simulink model "PILnewH"  (R2021a)
settings: Solver=FixedStepAuto  StartTime=0.0  StopTime=41.24  FixedStep=0.001  RelTol=1e-3  EnableMultiTasking=on
values from neighbouring files (symbols this model uses):
  den_lpf_d = den_lpf20    [Mainframe_init.m]    (also in load_autopilot.m)
  Emulated_FCC_IO_Delay = 7    [Mainframe_init.m]
  Enable_Gyros = 0    [Mainframe_init.m]
  Enable_INS = 0    [Mainframe_init.m]
  num_lpf_d = num_lpf20    [Mainframe_init.m]    (also in load_autopilot.m)
undefined symbols (not defined in the file or in its folder): act_dmp, act_omega, Actuator, Aerodynamics, aMode, Autopilot, AUX, c_b_WGS, c_be, c_flat, c_grav, c_h_geop0, c_h_geope, c_pa0, c_pe, c_r0, c_rot, c_rsma, c_Tmp0, d_siB_0, d_siB_max, d_siB_min, dd_siB_max, dd_siB_min, dev, DiscIntNeverNeededParam, e_pa, e_Tmp, Earth, fin_maxrate, flag_I_act_switch, flag_I_aero_switch, flag_I_flat, flag_I_gravity_switch, flag_I_rot, hcr, HIL_Data, JMMM_0, JMMM_e, JSPB_e, lat_0, lon_0, Mass_Props, mB_0, mM_0, mM_e, National_Instruments, pBII_0, PCIe, pMPB, pNPB, propellant_kg, prp_FBPB, prp_mdot, prp_T, pSPB, pwm_output1, qEG_0, qIB_0, qIE_0 ... (+29)
libraries: simulink x31, simulink_extras x24, aerolibcommonsys x4, px4lib x2, custom_blocks x1, pil_lib x1, aerolibtransform2 x1, sldrtlib x1, aerolibnav x1
(part 7 of 15)

== system PILnewH/Non-linear Flight Dynamic Model/Extract States/Assemble_States_Bus1/Three-axis Inertial Measurement Unit3/Three-axis Accelerometer/w x (w x d) ==
  "p q r " : Inport
  distance : Inport  Port=2
  w x (w x d) : Subsystem  mask(CrossProduct){aMode=aMode}
      mask help: shared_aeroblks:sharedaeroblkutil:blockCrossProductDesc
      mask init:
      | if aerosharedtest(gcb)
      |     aerosharedicon('shared');
      | else
      |     sharedautoicon('shared');
      | end
      mask Help: eval('if license(''test'',''Aerospace_Blockset'')aerosharedhelp(''threebythree_cross_product'');elseif license(''test'',''Powertrain_Blockset'')sharedautohelp(''threebythree_cross_product'');end')
      mask Display:
      | text(.5,.5,'Cross\nProduct\nC = AxB', ...
      | 	'HorizontalAlignment','Center',...
      | 	'VerticalAlignment','middle')
  w x d : Subsystem  mask(CrossProduct){aMode=aMode}
      mask help: shared_aeroblks:sharedaeroblkutil:blockCrossProductDesc
      mask init:
      | if aerosharedtest(gcb)
      |     aerosharedicon('shared');
      | else
      |     sharedautoicon('shared');
      | end
      mask Help: eval('if license(''test'',''Aerospace_Blockset'')aerosharedhelp(''threebythree_cross_product'');elseif license(''test'',''Powertrain_Blockset'')sharedautohelp(''threebythree_cross_product'');end')
      mask Display:
      | text(.5,.5,'Cross\nProduct\nC = AxB', ...
      | 	'HorizontalAlignment','Center',...
      | 	'VerticalAlignment','middle')
  w x ( w x d) : Outport  VectorParamsAs1DForOutWhenUnconnected=off
  wires:
  "p q r "/1 -> w x (w x d)/1(A), w x d/1(A)
  w x d/1(C) -> w x (w x d)/2(B)
  distance/1 -> w x d/2(B)
  w x (w x d)/1(C) -> w x ( w x d)/1

== system PILnewH/Non-linear Flight Dynamic Model/Extract States/Assemble_States_Bus1/Three-axis Inertial Measurement Unit3/Three-axis Accelerometer/wdot x d ==
  A : Inport
  B : Inport  Port=2
  "A " : InportShadow
  "B " : InportShadow  Port=2
  Subsystem : Subsystem
  Subsystem1 : Subsystem
  Sum : Sum  Inputs=+|-  InputSameDT=on  SaturateOnIntegerOverflow=on  OutDataTypeStr=Inherit: Same as first input
  C : Outport  VectorParamsAs1DForOutWhenUnconnected=off
  wires:
  Subsystem1/1(Out1) -> Sum/2
  Subsystem/1(Out1) -> Sum/1
  A/1 -> Subsystem/1(A)
  B/1 -> Subsystem/2(B)
  Sum/1 -> C/1
  "A "/1 -> Subsystem1/1(A)
  "B "/1 -> Subsystem1/2(B)

== system PILnewH/Non-linear Flight Dynamic Model/Extract States/Assemble_States_Bus1/Three-axis Inertial Measurement Unit3/Three-axis Gyroscope/Dynamics ==
  p q r : Inport
  Constant : Constant  Value=dtype_g
  No Dynamics : Subsystem
  Second-order Dynamics : Subsystem  mask(ContinuousFilter){wn=w_g, zn=z_g}
      mask prompts: wn "Natural frequency:"; zn "Damping ratio:"
      mask init:
      | aeroicon('aeroblk');
  Switch : Switch  Threshold=0.5
  "p q r " : Outport  VectorParamsAs1DForOutWhenUnconnected=off
  wires:
  p q r/1 -> Second-order Dynamics/1(In), No Dynamics/1(In1)
  No Dynamics/1(Out1) -> Switch/3
  Second-order Dynamics/1(Out) -> Switch/1
  Switch/1 -> "p q r "/1
  Constant/1 -> Switch/2

== system PILnewH/Non-linear Flight Dynamic Model/GRM_Airframe/aerodynamics/aerodynamic_via_lookup/calc_aero_coefficients/CLL_TLU ==
  alpha_deg : Inport
  beta_deg : Inport  Port=2
  dele_deg : Inport  Port=3
  dela_deg : Inport  Port=4
  delr_deg : Inport  Port=5
  p_ND_rps : Inport  Port=6
  1-D Lookup Table : Lookup_n-D  NumberOfTableDimensions=1  BreakpointsForDimension1=Aerodynamics.alpha_bkpts_ind1  Table=Aerodynamics.CLL_alpha  ExtrapMethod=Clip  UseLastTableValue=on  InternalRulePriority=Speed  RndMeth=Simplest  InputSameDT=on
      settings: AttributesFormatString=|
      | %<Table>
      | %<BreakpointsForDimension1>
  1-D Lookup Table1 : Lookup_n-D  NumberOfTableDimensions=1  BreakpointsForDimension1=Aerodynamics.beta_bkpts_ind1  Table=Aerodynamics.CLL_beta  ExtrapMethod=Clip  UseLastTableValue=on  InternalRulePriority=Speed  RndMeth=Simplest  InputSameDT=on
      settings: AttributesFormatString=|
      | %<Table>
      | %<BreakpointsForDimension1>
  2-D Lookup Table : Lookup_n-D  BreakpointsForDimension1=Aerodynamics.dele_inc_bkpts_ind1  BreakpointsForDimension2=Aerodynamics.dele_inc_bkpts_ind2  Table=Aerodynamics.CLL_dele_inc  ExtrapMethod=Clip  UseLastTableValue=on  InternalRulePriority=Speed  RndMeth=Simplest  InputSameDT=on
      settings: InputPortMap=u0,u1
      settings: AttributesFormatString=|
      | %<Table>
      | %<BreakpointsForDimension1>
      | %<BreakpointsForDimension2>
  2-D Lookup Table1 : Lookup_n-D  BreakpointsForDimension1=Aerodynamics.dela_inc_bkpts_ind1  BreakpointsForDimension2=Aerodynamics.dela_inc_bkpts_ind2  Table=Aerodynamics.CLL_dela_inc  ExtrapMethod=Clip  UseLastTableValue=on  InternalRulePriority=Speed  RndMeth=Simplest  InputSameDT=on
      settings: InputPortMap=u0,u1
      settings: AttributesFormatString=|
      | %<Table>
      | %<BreakpointsForDimension1>
      | %<BreakpointsForDimension2>
  2-D Lookup Table2 : Lookup_n-D  BreakpointsForDimension1=Aerodynamics.delr_inc_bkpts_ind1  BreakpointsForDimension2=Aerodynamics.delr_inc_bkpts_ind2  Table=Aerodynamics.CLL_delr_inc  ExtrapMethod=Clip  UseLastTableValue=on  InternalRulePriority=Speed  RndMeth=Simplest  InputSameDT=on
      settings: InputPortMap=u0,u1
      settings: AttributesFormatString=|
      | %<Table>
      | %<BreakpointsForDimension1>
      | %<BreakpointsForDimension2>
  Constant : Constant  Value=Aerodynamics.CLL_bias
      settings: AttributesFormatString=%<Value>
  Gain : Gain  Gain=Aerodynamics.CLL_scale
      settings: AttributesFormatString=%<Gain>
  Gain2 : Gain  Gain=Aerodynamics.CLL_p
      settings: AttributesFormatString=%<Gain>
  Sum1 : Sum  Inputs=+++++
  Sum2 : Sum
  Sum3 : Sum  Inputs=|++
  alpha_deg D1 : InportShadow
  alpha_deg D2 : InportShadow
  beta_deg D1 : InportShadow  Port=2
  CLL : Outport
  wires:
  p_ND_rps/1 -> Gain2/1
  Gain2/1 -> Sum1/5
  Gain/1 -> Sum3/1
  2-D Lookup Table2/1 -> Sum1/4  "CLL_delr"
  1-D Lookup Table/1 -> Sum2/1
  2-D Lookup Table1/1 -> Sum1/3  "CLL_dela"
  beta_deg/1 -> 1-D Lookup Table1/1
  1-D Lookup Table1/1 -> Sum2/2
  2-D Lookup Table/1 -> Sum1/2  "CLL_dele"
  dele_deg/1 -> 2-D Lookup Table/2
  alpha_deg D1/1 -> 2-D Lookup Table/1
  beta_deg D1/1 -> 2-D Lookup Table2/1
  dela_deg/1 -> 2-D Lookup Table1/2
  alpha_deg/1 -> 1-D Lookup Table/1
  alpha_deg D2/1 -> 2-D Lookup Table1/1
  delr_deg/1 -> 2-D Lookup Table2/2
  Sum2/1 -> Sum1/1  "CLL_0"
  Constant/1 -> Sum3/2
  Sum1/1 -> Gain/1
  Sum3/1 -> CLL/1  "CLL_B"

== system PILnewH/Non-linear Flight Dynamic Model/GRM_Airframe/aerodynamics/aerodynamic_via_lookup/calc_aero_coefficients/CLM_TLU ==
  alpha_deg : Inport
  beta_deg : Inport  Port=2
  dele_deg : Inport  Port=3
  dela_deg : Inport  Port=4
  delr_deg : Inport  Port=5
  q_ND_rps : Inport  Port=6
  1-D Lookup Table : Lookup_n-D  NumberOfTableDimensions=1  BreakpointsForDimension1=Aerodynamics.alpha_bkpts_ind1  Table=Aerodynamics.CLM_alpha  ExtrapMethod=Clip  UseLastTableValue=on  InternalRulePriority=Speed  RndMeth=Simplest  InputSameDT=on
      settings: AttributesFormatString=|
      | %<Table>
      | %<BreakpointsForDimension1>
  1-D Lookup Table1 : Lookup_n-D  NumberOfTableDimensions=1  BreakpointsForDimension1=Aerodynamics.beta_bkpts_ind1  Table=Aerodynamics.CLM_beta  ExtrapMethod=Clip  UseLastTableValue=on  InternalRulePriority=Speed  RndMeth=Simplest  InputSameDT=on
      settings: AttributesFormatString=|
      | %<Table>
      | %<BreakpointsForDimension1>
  2-D Lookup Table : Lookup_n-D  BreakpointsForDimension1=Aerodynamics.dele_inc_bkpts_ind1  BreakpointsForDimension2=Aerodynamics.dele_inc_bkpts_ind2  Table=Aerodynamics.CLM_dele_inc  ExtrapMethod=Clip  UseLastTableValue=on  InternalRulePriority=Speed  RndMeth=Simplest  InputSameDT=on
      settings: InputPortMap=u0,u1
      settings: AttributesFormatString=|
      | %<Table>
      | %<BreakpointsForDimension1>
      | %<BreakpointsForDimension2>
  2-D Lookup Table1 : Lookup_n-D  BreakpointsForDimension1=Aerodynamics.dela_inc_bkpts_ind1  BreakpointsForDimension2=Aerodynamics.dela_inc_bkpts_ind2  Table=Aerodynamics.CLM_dela_inc  ExtrapMethod=Clip  UseLastTableValue=on  InternalRulePriority=Speed  RndMeth=Simplest  InputSameDT=on
      settings: InputPortMap=u0,u1
      settings: AttributesFormatString=|
      | %<Table>
      | %<BreakpointsForDimension1>
      | %<BreakpointsForDimension2>
  2-D Lookup Table2 : Lookup_n-D  BreakpointsForDimension1=Aerodynamics.delr_inc_bkpts_ind1  BreakpointsForDimension2=Aerodynamics.delr_inc_bkpts_ind2  Table=Aerodynamics.CLM_delr_inc  ExtrapMethod=Clip  UseLastTableValue=on  InternalRulePriority=Speed  RndMeth=Simplest  InputSameDT=on
      settings: InputPortMap=u0,u1
      settings: AttributesFormatString=|
      | %<Table>
      | %<BreakpointsForDimension1>
      | %<BreakpointsForDimension2>
  Constant : Constant  Value=Aerodynamics.CLM_bias
      settings: AttributesFormatString=%<Value>
  Gain : Gain  Gain=Aerodynamics.CLM_scale
      settings: AttributesFormatString=%<Gain>
  Gain2 : Gain  Gain=Aerodynamics.CLM_q
      settings: AttributesFormatString=%<Gain>
  Sum1 : Sum  Inputs=+++++
  Sum2 : Sum
  Sum3 : Sum  Inputs=|++
  alpha_deg D1 : InportShadow
  alpha_deg D2 : InportShadow
  beta_deg D1 : InportShadow  Port=2
  CLM : Outport
  wires:
  q_ND_rps/1 -> Gain2/1
  Gain2/1 -> Sum1/5
  Sum3/1 -> CLM/1  "CLM_B"
  delr_deg/1 -> 2-D Lookup Table2/2
  alpha_deg D2/1 -> 2-D Lookup Table1/1
  dela_deg/1 -> 2-D Lookup Table1/2
  alpha_deg/1 -> 1-D Lookup Table/1
  beta_deg D1/1 -> 2-D Lookup Table2/1
  alpha_deg D1/1 -> 2-D Lookup Table/1
  1-D Lookup Table1/1 -> Sum2/2
  dele_deg/1 -> 2-D Lookup Table/2
  2-D Lookup Table/1 -> Sum1/2  "CLM_dele"
  2-D Lookup Table1/1 -> Sum1/3  "CLM_dela"
  beta_deg/1 -> 1-D Lookup Table1/1
  2-D Lookup Table2/1 -> Sum1/4  "CLM_delr"
  Sum2/1 -> Sum1/1  "CLM_0"
  1-D Lookup Table/1 -> Sum2/1
  Sum1/1 -> Gain/1
  Constant/1 -> Sum3/2
  Gain/1 -> Sum3/1

== system PILnewH/Non-linear Flight Dynamic Model/GRM_Airframe/aerodynamics/aerodynamic_via_lookup/calc_aero_coefficients/CLN_TLU ==
  alpha_deg : Inport
  beta_deg : Inport  Port=2
  dele_deg : Inport  Port=3
  dela_deg : Inport  Port=4
  delr_deg : Inport  Port=5
  r_ND_rps : Inport  Port=6
  1-D Lookup Table : Lookup_n-D  NumberOfTableDimensions=1  BreakpointsForDimension1=Aerodynamics.alpha_bkpts_ind1  Table=Aerodynamics.CLN_alpha  ExtrapMethod=Clip  UseLastTableValue=on  InternalRulePriority=Speed  RndMeth=Simplest  InputSameDT=on
      settings: AttributesFormatString=|
      | %<Table>
      | %<BreakpointsForDimension1>
  1-D Lookup Table1 : Lookup_n-D  NumberOfTableDimensions=1  BreakpointsForDimension1=Aerodynamics.beta_bkpts_ind1  Table=Aerodynamics.CLN_beta  ExtrapMethod=Clip  UseLastTableValue=on  InternalRulePriority=Speed  RndMeth=Simplest  InputSameDT=on
      settings: AttributesFormatString=|
      | %<Table>
      | %<BreakpointsForDimension1>
  2-D Lookup Table : Lookup_n-D  BreakpointsForDimension1=Aerodynamics.dele_inc_bkpts_ind1  BreakpointsForDimension2=Aerodynamics.dele_inc_bkpts_ind2  Table=Aerodynamics.CLN_dele_inc  ExtrapMethod=Clip  UseLastTableValue=on  InternalRulePriority=Speed  RndMeth=Simplest  InputSameDT=on
      settings: InputPortMap=u0,u1
      settings: AttributesFormatString=|
      | %<Table>
      | %<BreakpointsForDimension1>
      | %<BreakpointsForDimension2>
  2-D Lookup Table1 : Lookup_n-D  BreakpointsForDimension1=Aerodynamics.dela_inc_bkpts_ind1  BreakpointsForDimension2=Aerodynamics.dela_inc_bkpts_ind2  Table=Aerodynamics.CLN_dela_inc  ExtrapMethod=Clip  UseLastTableValue=on  InternalRulePriority=Speed  RndMeth=Simplest  InputSameDT=on
      settings: InputPortMap=u0,u1
      settings: AttributesFormatString=|
      | %<Table>
      | %<BreakpointsForDimension1>
      | %<BreakpointsForDimension2>
  2-D Lookup Table2 : Lookup_n-D  BreakpointsForDimension1=Aerodynamics.delr_inc_bkpts_ind1  BreakpointsForDimension2=Aerodynamics.delr_inc_bkpts_ind2  Table=Aerodynamics.CLN_delr_inc  ExtrapMethod=Clip  UseLastTableValue=on  InternalRulePriority=Speed  RndMeth=Simplest  InputSameDT=on
      settings: InputPortMap=u0,u1
      settings: AttributesFormatString=|
      | %<Table>
      | %<BreakpointsForDimension1>
      | %<BreakpointsForDimension2>
  Constant : Constant  Value=Aerodynamics.CLN_bias
      settings: AttributesFormatString=%<Value>
  Gain : Gain  Gain=Aerodynamics.CLN_scale
      settings: AttributesFormatString=%<Gain>
  Gain2 : Gain  Gain=Aerodynamics.CLN_r
      settings: AttributesFormatString=%<Gain>
  Sum1 : Sum  Inputs=+++++
  Sum2 : Sum
  Sum3 : Sum  Inputs=|++
  alpha_deg D1 : InportShadow
  alpha_deg D2 : InportShadow
  beta_deg D1 : InportShadow  Port=2
  CLN : Outport
  wires:
  r_ND_rps/1 -> Gain2/1
  Sum3/1 -> CLN/1  "CLN_B"
  beta_deg/1 -> 1-D Lookup Table1/1
  1-D Lookup Table/1 -> Sum2/1
  2-D Lookup Table2/1 -> Sum1/4  "CLN_delr"
  Sum2/1 -> Sum1/1  "CLN_0"
  alpha_deg D1/1 -> 2-D Lookup Table/1
  beta_deg D1/1 -> 2-D Lookup Table2/1
  dele_deg/1 -> 2-D Lookup Table/2
  alpha_deg D2/1 -> 2-D Lookup Table1/1
  2-D Lookup Table1/1 -> Sum1/3  "CLN_dela"
  alpha_deg/1 -> 1-D Lookup Table/1
  dela_deg/1 -> 2-D Lookup Table1/2
  Gain2/1 -> Sum1/5
  1-D Lookup Table1/1 -> Sum2/2
  delr_deg/1 -> 2-D Lookup Table2/2
  2-D Lookup Table/1 -> Sum1/2  "CLN_dele"
  Sum1/1 -> Gain/1
  Constant/1 -> Sum3/2
  Gain/1 -> Sum3/1

== system PILnewH/Non-linear Flight Dynamic Model/GRM_Airframe/aerodynamics/aerodynamic_via_lookup/calc_aero_coefficients/CX_TLU ==
  alpha_deg : Inport
  beta_deg : Inport  Port=2
  dele_deg : Inport  Port=3
  dela_deg : Inport  Port=4
  delr_deg : Inport  Port=5
  2-D Lookup Table : Lookup_n-D  BreakpointsForDimension1=Aerodynamics.alpha_beta_bkpts_ind1  BreakpointsForDimension2=Aerodynamics.alpha_beta_bkpts_ind2  Table=Aerodynamics.CX_alpha_beta  ExtrapMethod=Clip  UseLastTableValue=on  InternalRulePriority=Speed  RndMeth=Simplest  InputSameDT=on
      settings: InputPortMap=u0,u1
      settings: AttributesFormatString=|
      | %<Table>
      | %<BreakpointsForDimension1>
      | %<BreakpointsForDimension2>
  2-D Lookup Table1 : Lookup_n-D  BreakpointsForDimension1=Aerodynamics.dele_inc_bkpts_ind1  BreakpointsForDimension2=Aerodynamics.dele_inc_bkpts_ind2  Table=Aerodynamics.CX_dele_inc  ExtrapMethod=Clip  UseLastTableValue=on  InternalRulePriority=Speed  RndMeth=Simplest  InputSameDT=on
      settings: InputPortMap=u0,u1
      settings: AttributesFormatString=|
      | %<Table>
      | %<BreakpointsForDimension1>
      | %<BreakpointsForDimension2>
  2-D Lookup Table2 : Lookup_n-D  BreakpointsForDimension1=Aerodynamics.dela_inc_bkpts_ind1  BreakpointsForDimension2=Aerodynamics.dela_inc_bkpts_ind2  Table=Aerodynamics.CX_dela_inc  ExtrapMethod=Clip  UseLastTableValue=on  InternalRulePriority=Speed  RndMeth=Simplest  InputSameDT=on
      settings: InputPortMap=u0,u1
      settings: AttributesFormatString=|
      | %<Table>
      | %<BreakpointsForDimension1>
      | %<BreakpointsForDimension2>
  2-D Lookup Table3 : Lookup_n-D  BreakpointsForDimension1=Aerodynamics.delr_inc_bkpts_ind1  BreakpointsForDimension2=Aerodynamics.delr_inc_bkpts_ind2  Table=Aerodynamics.CX_delr_inc  ExtrapMethod=Clip  UseLastTableValue=on  InternalRulePriority=Speed  RndMeth=Simplest  InputSameDT=on
      settings: InputPortMap=u0,u1
      settings: AttributesFormatString=|
      | %<Table>
      | %<BreakpointsForDimension1>
      | %<BreakpointsForDimension2>
  Constant : Constant  Value=Aerodynamics.CX_bias
      settings: AttributesFormatString=%<Value>
  Gain : Gain  Gain=Aerodynamics.CX_scale
      settings: AttributesFormatString=%<Gain>
  Sum : Sum  Inputs=++++
  Sum1 : Sum  Inputs=|++
  alpha_deg D1 : InportShadow
  alpha_deg D2 : InportShadow
  beta_deg D1 : InportShadow  Port=2
  CX : Outport
  wires:
  Sum/1 -> Gain/1
  2-D Lookup Table1/1 -> Sum/2  "CX_dele"
  2-D Lookup Table2/1 -> Sum/3  "CX_dela"
  2-D Lookup Table/1 -> Sum/1  "CX_0"
  alpha_deg/1 -> 2-D Lookup Table/1
  beta_deg/1 -> 2-D Lookup Table/2
  alpha_deg D1/1 -> 2-D Lookup Table1/1
  dele_deg/1 -> 2-D Lookup Table1/2
  dela_deg/1 -> 2-D Lookup Table2/2
  2-D Lookup Table3/1 -> Sum/4  "CX_delr"
  delr_deg/1 -> 2-D Lookup Table3/2
  alpha_deg D2/1 -> 2-D Lookup Table2/1
  beta_deg D1/1 -> 2-D Lookup Table3/1
  Constant/1 -> Sum1/2
  Gain/1 -> Sum1/1
  Sum1/1 -> CX/1  "CX_B"

== system PILnewH/Non-linear Flight Dynamic Model/GRM_Airframe/aerodynamics/aerodynamic_via_lookup/calc_aero_coefficients/CY_TLU ==
  alpha_deg : Inport
  beta_deg : Inport  Port=2
  dele_deg : Inport  Port=3
  dela_deg : Inport  Port=4
  delr_deg : Inport  Port=5
  1-D Lookup Table : Lookup_n-D  NumberOfTableDimensions=1  BreakpointsForDimension1=Aerodynamics.alpha_bkpts_ind1  Table=Aerodynamics.CY_alpha  ExtrapMethod=Clip  UseLastTableValue=on  InternalRulePriority=Speed  RndMeth=Simplest  InputSameDT=on
      settings: AttributesFormatString=|
      | %<Table>
      | %<BreakpointsForDimension1>
  1-D Lookup Table1 : Lookup_n-D  NumberOfTableDimensions=1  BreakpointsForDimension1=Aerodynamics.beta_bkpts_ind1  Table=Aerodynamics.CY_beta  ExtrapMethod=Clip  UseLastTableValue=on  InternalRulePriority=Speed  RndMeth=Simplest  InputSameDT=on
      settings: AttributesFormatString=|
      | %<Table>
      | %<BreakpointsForDimension1>
  2-D Lookup Table : Lookup_n-D  BreakpointsForDimension1=Aerodynamics.dele_inc_bkpts_ind1  BreakpointsForDimension2=Aerodynamics.dele_inc_bkpts_ind2  Table=Aerodynamics.CY_dele_inc  ExtrapMethod=Clip  UseLastTableValue=on  InternalRulePriority=Speed  RndMeth=Simplest  InputSameDT=on
      settings: InputPortMap=u0,u1
      settings: AttributesFormatString=|
      | %<Table>
      | %<BreakpointsForDimension1>
      | %<BreakpointsForDimension2>
  2-D Lookup Table1 : Lookup_n-D  BreakpointsForDimension1=Aerodynamics.dela_inc_bkpts_ind1  BreakpointsForDimension2=Aerodynamics.dela_inc_bkpts_ind2  Table=Aerodynamics.CY_dela_inc  ExtrapMethod=Clip  UseLastTableValue=on  InternalRulePriority=Speed  RndMeth=Simplest  InputSameDT=on
      settings: InputPortMap=u0,u1
      settings: AttributesFormatString=|
      | %<Table>
      | %<BreakpointsForDimension1>
      | %<BreakpointsForDimension2>
  2-D Lookup Table2 : Lookup_n-D  BreakpointsForDimension1=Aerodynamics.delr_inc_bkpts_ind1  BreakpointsForDimension2=Aerodynamics.delr_inc_bkpts_ind2  Table=Aerodynamics.CY_delr_inc  ExtrapMethod=Clip  UseLastTableValue=on  InternalRulePriority=Speed  RndMeth=Simplest  InputSameDT=on
      settings: InputPortMap=u0,u1
      settings: AttributesFormatString=|
      | %<Table>
      | %<BreakpointsForDimension1>
      | %<BreakpointsForDimension2>
  Constant : Constant  Value=Aerodynamics.CY_bias
      settings: AttributesFormatString=%<Value>
  Gain : Gain  Gain=Aerodynamics.CY_scale
      settings: AttributesFormatString=%<Gain>
  Sum : Sum  Inputs=++++
  Sum1 : Sum
  Sum2 : Sum  Inputs=|++
  alpha_deg D1 : InportShadow
  alpha_deg D2 : InportShadow
  beta_deg D1 : InportShadow  Port=2
  CY : Outport
  wires:
  Sum2/1 -> CY/1  "CY_B"
  beta_deg/1 -> 1-D Lookup Table1/1
  1-D Lookup Table/1 -> Sum1/1
  1-D Lookup Table1/1 -> Sum1/2
  alpha_deg/1 -> 1-D Lookup Table/1
  alpha_deg D1/1 -> 2-D Lookup Table/1
  alpha_deg D2/1 -> 2-D Lookup Table1/1
  2-D Lookup Table2/1 -> Sum/4  "CY_delr"
  delr_deg/1 -> 2-D Lookup Table2/2
  2-D Lookup Table1/1 -> Sum/3  "CY_dela"
  2-D Lookup Table/1 -> Sum/2  "CY_dele"
  beta_deg D1/1 -> 2-D Lookup Table2/1
  dela_deg/1 -> 2-D Lookup Table1/2
  dele_deg/1 -> 2-D Lookup Table/2
  Sum1/1 -> Sum/1  "CY_0"
  Gain/1 -> Sum2/1
  Constant/1 -> Sum2/2
  Sum/1 -> Gain/1

== system PILnewH/Non-linear Flight Dynamic Model/GRM_Airframe/aerodynamics/aerodynamic_via_lookup/calc_aero_coefficients/CZ_TLU ==
  alpha_deg : Inport
  beta_deg : Inport  Port=2
  dele_deg : Inport  Port=3
  dela_deg : Inport  Port=4
  delr_deg : Inport  Port=5
  1-D Lookup Table : Lookup_n-D  NumberOfTableDimensions=1  BreakpointsForDimension1=Aerodynamics.alpha_bkpts_ind1  Table=Aerodynamics.CZ_alpha  ExtrapMethod=Clip  UseLastTableValue=on  InternalRulePriority=Speed  RndMeth=Simplest  InputSameDT=on
      settings: AttributesFormatString=|
      | %<Table>
      | %<BreakpointsForDimension1>
  1-D Lookup Table1 : Lookup_n-D  NumberOfTableDimensions=1  BreakpointsForDimension1=Aerodynamics.beta_bkpts_ind1  Table=Aerodynamics.CZ_beta  ExtrapMethod=Clip  UseLastTableValue=on  InternalRulePriority=Speed  RndMeth=Simplest  InputSameDT=on
      settings: AttributesFormatString=|
      | %<Table>
      | %<BreakpointsForDimension1>
  2-D Lookup Table : Lookup_n-D  BreakpointsForDimension1=Aerodynamics.dele_inc_bkpts_ind1  BreakpointsForDimension2=Aerodynamics.dele_inc_bkpts_ind2  Table=Aerodynamics.CZ_dele_inc  ExtrapMethod=Clip  UseLastTableValue=on  InternalRulePriority=Speed  RndMeth=Simplest  InputSameDT=on
      settings: InputPortMap=u0,u1
      settings: AttributesFormatString=|
      | %<Table>
      | %<BreakpointsForDimension1>
      | %<BreakpointsForDimension2>
  2-D Lookup Table1 : Lookup_n-D  BreakpointsForDimension1=Aerodynamics.dela_inc_bkpts_ind1  BreakpointsForDimension2=Aerodynamics.dela_inc_bkpts_ind2  Table=Aerodynamics.CZ_dela_inc  ExtrapMethod=Clip  UseLastTableValue=on  InternalRulePriority=Speed  RndMeth=Simplest  InputSameDT=on
      settings: InputPortMap=u0,u1
      settings: AttributesFormatString=|
      | %<Table>
      | %<BreakpointsForDimension1>
      | %<BreakpointsForDimension2>
  2-D Lookup Table2 : Lookup_n-D  BreakpointsForDimension1=Aerodynamics.delr_inc_bkpts_ind1  BreakpointsForDimension2=Aerodynamics.delr_inc_bkpts_ind2  Table=Aerodynamics.CZ_delr_inc  ExtrapMethod=Clip  UseLastTableValue=on  InternalRulePriority=Speed  RndMeth=Simplest  InputSameDT=on
      settings: InputPortMap=u0,u1
      settings: AttributesFormatString=|
      | %<Table>
      | %<BreakpointsForDimension1>
      | %<BreakpointsForDimension2>
  Constant : Constant  Value=Aerodynamics.CZ_bias
      settings: AttributesFormatString=%<Value>
  Gain : Gain  Gain=Aerodynamics.CZ_scale
      settings: AttributesFormatString=%<Gain>
  Sum : Sum  Inputs=++++
  Sum1 : Sum
  Sum2 : Sum  Inputs=|++
  alpha_deg D1 : InportShadow
  alpha_deg D2 : InportShadow
  beta_deg D1 : InportShadow  Port=2
  CZ : Outport
  wires:
  dele_deg/1 -> 2-D Lookup Table/2
  dela_deg/1 -> 2-D Lookup Table1/2
  beta_deg D1/1 -> 2-D Lookup Table2/1
  2-D Lookup Table/1 -> Sum/2  "CZ_dele"
  2-D Lookup Table1/1 -> Sum/3  "CZ_dela"
  delr_deg/1 -> 2-D Lookup Table2/2
  2-D Lookup Table2/1 -> Sum/4  "CZ_delr"
  alpha_deg D2/1 -> 2-D Lookup Table1/1
  alpha_deg D1/1 -> 2-D Lookup Table/1
  alpha_deg/1 -> 1-D Lookup Table/1
  1-D Lookup Table1/1 -> Sum1/2
  1-D Lookup Table/1 -> Sum1/1
  Sum1/1 -> Sum/1  "CZ_0"
  beta_deg/1 -> 1-D Lookup Table1/1
  Sum2/1 -> CZ/1  "CZ_B"
  Constant/1 -> Sum2/2
  Gain/1 -> Sum2/1
  Sum/1 -> Gain/1

== system PILnewH/Non-linear Flight Dynamic Model/GRM_Airframe/aerodynamics/aerodynamic_via_lookup/calc_aero_for_mom/create_pAPB ==
  Constant : Constant  Value=Aerodynamics.xcg
      settings: AttributesFormatString=%<Value>
  Constant3 : Constant  Value=0
  Gain : Gain  Gain=-1
  Vector Concatenate : Concatenate  NumInputs=3
  pAPB : Outport  VectorParamsAs1DForOutWhenUnconnected=off
  wires:
  Constant3/1 -> Vector Concatenate/3, Vector Concatenate/2
  Gain/1 -> Vector Concatenate/1
  Constant/1 -> Gain/1
  Vector Concatenate/1 -> pAPB/1  "pAPB"

== system PILnewH/Non-linear Flight Dynamic Model/GRM_Airframe/aerodynamics/aerodynamic_via_lookup/calc_aero_for_mom/cross_product ==
  note: Outputs [size]:
      |
      | r1 x r2  [3x1]
  note: Inputs [size]:
      |
      | r1 [3x1]
      | r2 [3x1]
  r1 : Inport
  r2 : Inport  Port=2
  Demux2 : Demux  Outputs=[1;1;1]
      settings: DisplayOption=none
  Demux3 : Demux  Outputs=[1;1;1]
      settings: DisplayOption=none
  Product{2..7} (6 alike) : Product  InputSameDT=on  RndMeth=Zero  SaturateOnIntegerOverflow=on  OutDataTypeStr=Inherit: Same as first input
  Sum : Sum  Inputs=+-  InputSameDT=on  SaturateOnIntegerOverflow=on  OutDataTypeStr=Inherit: Same as first input
  Sum1 : Sum  Inputs=+-  InputSameDT=on  SaturateOnIntegerOverflow=on  OutDataTypeStr=Inherit: Same as first input
  Sum2 : Sum  Inputs=+-  InputSameDT=on  SaturateOnIntegerOverflow=on  OutDataTypeStr=Inherit: Same as first input
  Vector Concatenate : Concatenate  NumInputs=3
  r1_x_r2 : Outport  PortDimensions=[3,1]  VectorParamsAs1DForOutWhenUnconnected=off
  wires:
  Demux2/2 -> Product2/1, Product7/1
  Demux3/3 -> Product5/2, Product2/2
  Demux3/2 -> Product6/2, Product3/2
  Demux2/3 -> Product3/1, Product4/1
  Demux3/1 -> Product7/2, Product4/2
  Demux2/1 -> Product6/1, Product5/1
  Product2/1 -> Sum/1
  Product3/1 -> Sum/2
  Product4/1 -> Sum1/1
  Product5/1 -> Sum1/2
  Product6/1 -> Sum2/1
  Product7/1 -> Sum2/2
  Sum/1 -> Vector Concatenate/1
  Sum1/1 -> Vector Concatenate/2
  Sum2/1 -> Vector Concatenate/3
  r1/1 -> Demux2/1
  r2/1 -> Demux3/1
  Vector Concatenate/1 -> r1_x_r2/1

== system PILnewH/Non-linear Flight Dynamic Model/GRM_Airframe/aerodynamics/aerodynamic_via_lookup/calc_aero_for_mom/launch_rail ==
  hBE : Inport
  FBAB_c : Inport  Port=2
  Constant1 : Constant  Value=flag_I_aero_switch
  Constant3 : Constant  Value=0
  Subtract : Sum  Inputs=++-
  Switch : Switch  Criteria=u2 > Threshold  Threshold=0.05
  Vector Concatenate : Concatenate  NumInputs=3
  initial_altitude : Subsystem
  FBAB : Outport  VectorParamsAs1DForOutWhenUnconnected=off
  wires:
  Constant1/1 -> Subtract/2
  hBE/1 -> Subtract/1
  Subtract/1 -> Switch/2
  Constant3/1 -> Vector Concatenate/1, Vector Concatenate/2, Vector Concatenate/3
  Switch/1 -> FBAB/1  "FBAB"
  Vector Concatenate/1 -> Switch/3
  FBAB_c/1 -> Switch/1
  initial_altitude/1(hBE_0) -> Subtract/3

== system PILnewH/Non-linear Flight Dynamic Model/GRM_Airframe/aerodynamics/aerodynamic_via_lookup/calc_aero_for_mom/launch_rail1 ==
  hBE : Inport
  MBAB_c : Inport  Port=2
  Constant1 : Constant  Value=flag_I_aero_switch
  Constant3 : Constant  Value=0
  Subtract : Sum  Inputs=++-
  Switch : Switch  Criteria=u2 > Threshold  Threshold=0.05
  Vector Concatenate : Concatenate  NumInputs=3
  initial_altitude : Subsystem
  MBAB : Outport  VectorParamsAs1DForOutWhenUnconnected=off
  wires:
  initial_altitude/1(hBE_0) -> Subtract/3
  MBAB_c/1 -> Switch/1
  Vector Concatenate/1 -> Switch/3
  Switch/1 -> MBAB/1  "MBAB"
  Constant3/1 -> Vector Concatenate/3, Vector Concatenate/2, Vector Concatenate/1
  Subtract/1 -> Switch/2
  hBE/1 -> Subtract/1
  Constant1/1 -> Subtract/2

== system PILnewH/Non-linear Flight Dynamic Model/GRM_Airframe/environment/WGS84_Gravitation/WGS84_2_ECEF/WGS84 Transformation Parameter  ==
  phi : Inport
  Add2 : Sum  Inputs=+-
  Divide : Product  Inputs=**
  Divide1 : Product  Inputs=**
  Divide2 : Product  Inputs=**
  Divide3 : Product  Inputs=/*
  Sqrt : Sqrt  SaturateOnIntegerOverflow=on
  Subsystem : Subsystem
  Trigonometric Function : Trigonometry
  "WGS84 Semi-major Axis, [m]" : Constant  Value=c_rsma
  "WGS84 Semi-minor Axis, [m]" : Constant  Value=c_b_WGS
  a3 : Constant
  N : Outport  VectorParamsAs1DForOutWhenUnconnected=off
  e : Outport  Port=2  VectorParamsAs1DForOutWhenUnconnected=off
  wires:
  "WGS84 Semi-minor Axis, [m]"/1 -> Subsystem/1(b)  "c_b_WGS"
  "WGS84 Semi-major Axis, [m]"/1 -> Subsystem/2(a), Divide3/2  "c_rsma"
  Divide1/1 -> Divide2/1  "sin(phi)^2"
  Divide3/1 -> N/1  "N"
  Sqrt/1 -> Divide3/1
  a3/1 -> Add2/1
  Divide2/1 -> Add2/2
  Trigonometric Function/1 -> Divide1/2, Divide1/1
  Divide/1 -> Divide2/2  "e^2"
  Subsystem/1(e) -> e/1, Divide/2, Divide/1
  Add2/1 -> Sqrt/1
  phi/1 -> Trigonometric Function/1

== system PILnewH/Non-linear Flight Dynamic Model/GRM_Airframe/environment/atmosphere_static_ISO_2533/tmp_and_pressure_ISO_2533/static_Temperature ==
  Tmp_ref : Inport
  h_geop : Inport  Port=2
  h_geop_ref : Inport  Port=3
  Add : Sum
  Product : Product
  Subtract : Sum  Inputs=+-
  Tmp_gradient_tropo : Constant  Value=c_be
  Tmp : Outport  VectorParamsAs1DForOutWhenUnconnected=off
  wires:
  Subtract/1 -> Product/2
  Tmp_gradient_tropo/1 -> Product/1
  Product/1 -> Add/2
  Add/1 -> Tmp/1  "Tmp"
  Tmp_ref/1 -> Add/1
  h_geop/1 -> Subtract/1
  h_geop_ref/1 -> Subtract/2

== system PILnewH/Non-linear Flight Dynamic Model/GRM_Airframe/environment/atmosphere_static_ISO_2533/tmp_and_pressure_ISO_2533/static_pressure ==
  h_geop_ref : Inport
  h_geop : Inport  Port=2
  Tmp_ref : Inport  Port=3
  pa_ref : Inport  Port=4
  Add : Sum
  Constant1 : Constant
  Divide : Product  Inputs=*/*
  Math Function : Math  Operator=pow  SignedPower=on  SaturateOnIntegerOverflow=on
  Product : Product
  Subtract : Sum  Inputs=-+
  Tmp_gradient_tropo : Constant  Value=c_be
  pressure_exponent : Constant  Value=c_pe
  pa : Outport  VectorParamsAs1DForOutWhenUnconnected=off
  wires:
  pressure_exponent/1 -> Math Function/2
  h_geop/1 -> Subtract/2
  Divide/1 -> Add/2
  h_geop_ref/1 -> Subtract/1
  Tmp_ref/1 -> Divide/2
  Add/1 -> Math Function/1
  pa_ref/1 -> Product/2
  Math Function/1 -> Product/1
  Subtract/1 -> Divide/1
  Constant1/1 -> Add/1
  Product/1 -> pa/1  "pa"
  Tmp_gradient_tropo/1 -> Divide/3

== system PILnewH/Non-linear Flight Dynamic Model/GRM_Airframe/gravity/launch_rail/initial_altitude/trafo_E_to_geodetic ==
  note: Outputs [size]:
      |
      | geodetic longitude [1]
      | geodetic latitude [1]
      | geodetic altitude [1]
  note: Inputs [size]:
      |
      | position_E [3]
  pBEE : Inport
  Geodetic_altitude : Subsystem
  Geodetic_latitude : Subsystem
  Selector1 : Selector  IndexMode=Zero-based  InputPortWidth=3  IndexOptions=Index vector (dialog)  Indices=1  OutputSizes=1
  Selector2 : Selector  IndexMode=Zero-based  InputPortWidth=3  IndexOptions=Index vector (dialog)  Indices=0  OutputSizes=1
  Trigonometric Function1 : Trigonometry  Operator=atan2
  c_flat : Constant  Value=c_flat
  c_rsma : Constant  Value=c_rsma
  lon : Outport  VectorParamsAs1DForOutWhenUnconnected=off
  lat : Outport  Port=2  VectorParamsAs1DForOutWhenUnconnected=off
  alt : Outport  Port=3  VectorParamsAs1DForOutWhenUnconnected=off
  wires:
  c_flat/1 -> Geodetic_altitude/3(c_flat), Geodetic_latitude/3(c_flat)  "c_flat"
  c_rsma/1 -> Geodetic_latitude/2(c_rsma), Geodetic_altitude/2(c_rsma)  "c_rsma"
  Selector1/1 -> Trigonometric Function1/1  "pBEE_y"
  Selector2/1 -> Trigonometric Function1/2  "pBEE_x"
  Geodetic_latitude/1(lat) -> Geodetic_altitude/4(lat), lat/1
  Geodetic_altitude/1(alt) -> alt/1
  Trigonometric Function1/1 -> lon/1  "lon"
  pBEE/1 -> Selector1/1, Selector2/1, Geodetic_latitude/1(pBEE), Geodetic_altitude/1(pBEE)  "pBEE"

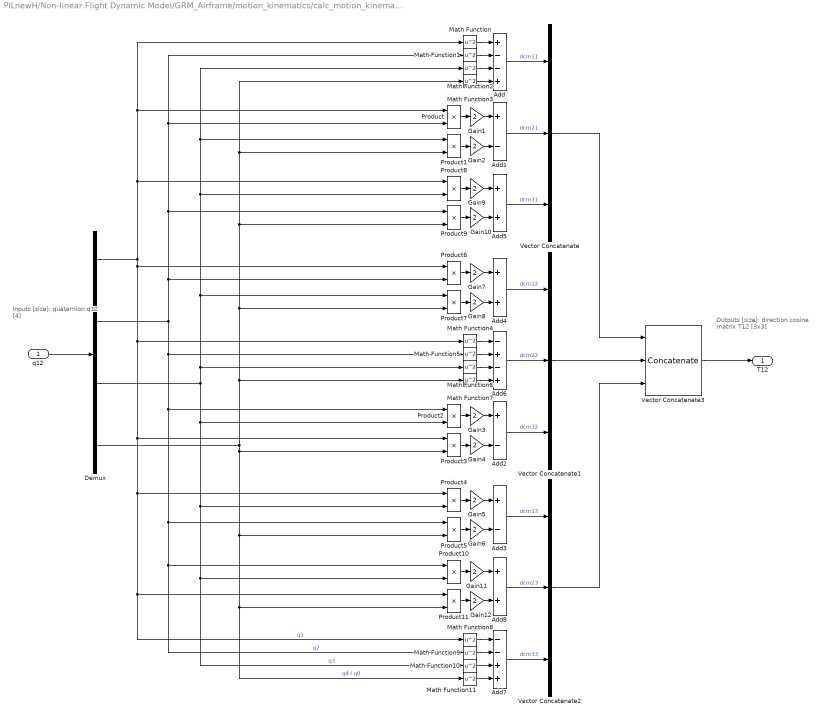
== system PILnewH/Non-linear Flight Dynamic Model/GRM_Airframe/motion_kinematics/calc_motion_kinematics/calc_transformation_matrix/T12_from_q1 ==
  note: Inputs [size]:
      |
      | quaternion q12 [4]
  note: Outputs [size]:
      |
      | direction cosine matrix T12 [3x3]
  q12 : Inport  PortDimensions=4
  Add : Sum  Inputs=+--+
  Add1 : Sum  Inputs=+-
  Add2 : Sum  Inputs=+-
  Add3 : Sum  Inputs=+-
  Add4 : Sum
  Add5 : Sum
  Add6 : Sum  Inputs=-+-+
  Add7 : Sum  Inputs=--++
  Add8 : Sum
  Demux : Demux
  Gain{1..12} (12 alike) : Gain  Gain=2
  Math Function{,1..11} (12 alike) : Math  Operator=square  SignedPower=on  SaturateOnIntegerOverflow=on
  Product{,1..11} (12 alike) : Product
  Vector Concatenate : Concatenate  NumInputs=3
  Vector Concatenate1 : Concatenate  NumInputs=3
  Vector Concatenate2 : Concatenate  NumInputs=3
  Vector Concatenate3 : Concatenate  NumInputs=3  Mode=Multidimensional array  ConcatenateDimension=2
  T12 : Outport  PortDimensions=[3 3]  VectorParamsAs1DForOutWhenUnconnected=off
  wires:
  Product10/1 -> Gain11/1
  Product11/1 -> Gain12/1
  Gain11/1 -> Add8/1
  Gain12/1 -> Add8/2
  Math Function8/1 -> Add7/1
  Math Function9/1 -> Add7/2
  Math Function11/1 -> Add7/4
  Math Function10/1 -> Add7/3
  Math Function4/1 -> Add6/1
  Math Function5/1 -> Add6/2
  Math Function7/1 -> Add6/4
  Math Function6/1 -> Add6/3
  Product8/1 -> Gain9/1
  Product9/1 -> Gain10/1
  Gain9/1 -> Add5/1
  Gain10/1 -> Add5/2
  Product6/1 -> Gain7/1
  Product7/1 -> Gain8/1
  Gain7/1 -> Add4/1
  Gain8/1 -> Add4/2
  Product4/1 -> Gain5/1
  Product5/1 -> Gain6/1
  Gain5/1 -> Add3/1
  Gain6/1 -> Add3/2
  Product2/1 -> Gain3/1
  Product3/1 -> Gain4/1
  Gain3/1 -> Add2/1
  Gain4/1 -> Add2/2
  Gain2/1 -> Add1/2
  Gain1/1 -> Add1/1
  Product1/1 -> Gain2/1
  Product/1 -> Gain1/1
  Math Function3/1 -> Add/4
  Math Function2/1 -> Add/3
  Math Function1/1 -> Add/2
  Math Function/1 -> Add/1
  Add7/1 -> Vector Concatenate2/3  "dcm33"
  Add8/1 -> Vector Concatenate2/2  "dcm23"
  Add3/1 -> Vector Concatenate2/1  "dcm13"
  Add2/1 -> Vector Concatenate1/3  "dcm32"
  Add6/1 -> Vector Concatenate1/2  "dcm22"
  Add4/1 -> Vector Concatenate1/1  "dcm12"
  Add5/1 -> Vector Concatenate/3  "dcm31"
  Add1/1 -> Vector Concatenate/2  "dcm21"
  Add/1 -> Vector Concatenate/1  "dcm11"
  Vector Concatenate1/1 -> Vector Concatenate3/2
  Vector Concatenate2/1 -> Vector Concatenate3/3
  Vector Concatenate/1 -> Vector Concatenate3/1
  Vector Concatenate3/1 -> T12/1
  Demux/4 -> Product3/2, Product11/2, Math Function11/1, Product5/2, Math Function3/1, Product1/2, Product9/2, Product7/2, Math Function7/1  "q4 / q0"
  Demux/3 -> Math Function2/1, Product1/1, Product8/2, Product7/1, Math Function6/1, Product10/2, Math Function10/1, Product4/2, Product2/2  "q3"
  Demux/2 -> Math Function1/1, Product/2, Product9/1, Product6/2, Math Function5/1, Math Function9/1, Product10/1, Product5/1, Product2/1  "q2"
  Demux/1 -> Product6/1, Math Function4/1, Math Function8/1, Product11/1, Product4/1, Product3/1, Math Function/1, Product/1, Product8/1  "q1"
  q12/1 -> Demux/1

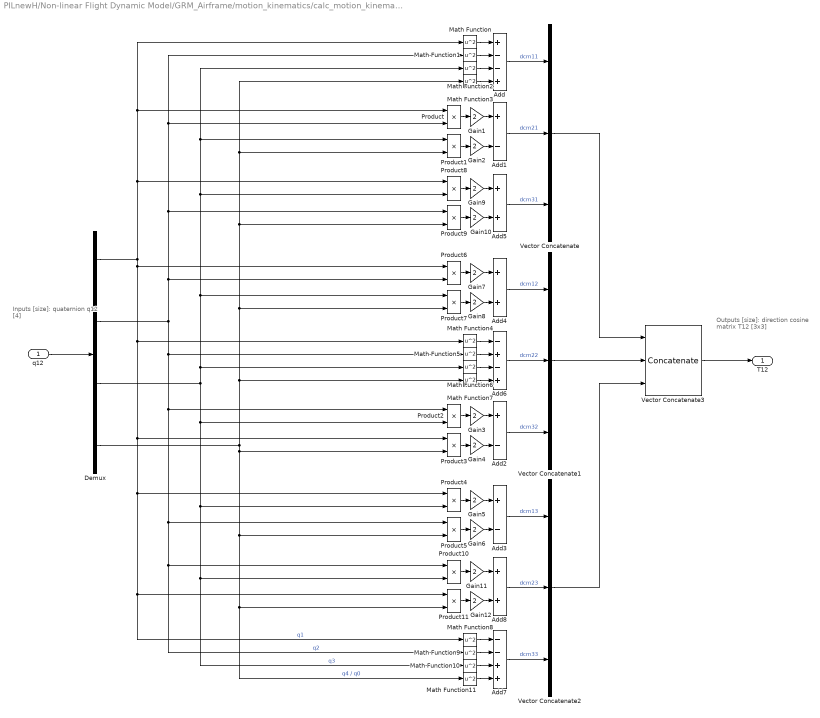
== system PILnewH/Non-linear Flight Dynamic Model/GRM_Airframe/motion_kinematics/calc_motion_kinematics/calc_transformation_matrix/T12_from_q12 ==
  note: Inputs [size]:
      |
      | quaternion q12 [4]
  note: Outputs [size]:
      |
      | direction cosine matrix T12 [3x3]
  q12 : Inport  PortDimensions=4
  Add : Sum  Inputs=+--+
  Add1 : Sum  Inputs=+-
  Add2 : Sum  Inputs=+-
  Add3 : Sum  Inputs=+-
  Add4 : Sum
  Add5 : Sum
  Add6 : Sum  Inputs=-+-+
  Add7 : Sum  Inputs=--++
  Add8 : Sum
  Demux : Demux
  Gain{1..12} (12 alike) : Gain  Gain=2
  Math Function{,1..11} (12 alike) : Math  Operator=square  SignedPower=on  SaturateOnIntegerOverflow=on
  Product{,1..11} (12 alike) : Product
  Vector Concatenate : Concatenate  NumInputs=3
  Vector Concatenate1 : Concatenate  NumInputs=3
  Vector Concatenate2 : Concatenate  NumInputs=3
  Vector Concatenate3 : Concatenate  NumInputs=3  Mode=Multidimensional array  ConcatenateDimension=2
  T12 : Outport  PortDimensions=[3 3]  VectorParamsAs1DForOutWhenUnconnected=off
  wires:
  Product10/1 -> Gain11/1
  Product11/1 -> Gain12/1
  Gain11/1 -> Add8/1
  Gain12/1 -> Add8/2
  Math Function8/1 -> Add7/1
  Math Function9/1 -> Add7/2
  Math Function11/1 -> Add7/4
  Math Function10/1 -> Add7/3
  Math Function4/1 -> Add6/1
  Math Function5/1 -> Add6/2
  Math Function7/1 -> Add6/4
  Math Function6/1 -> Add6/3
  Product8/1 -> Gain9/1
  Product9/1 -> Gain10/1
  Gain9/1 -> Add5/1
  Gain10/1 -> Add5/2
  Product6/1 -> Gain7/1
  Product7/1 -> Gain8/1
  Gain7/1 -> Add4/1
  Gain8/1 -> Add4/2
  Product4/1 -> Gain5/1
  Product5/1 -> Gain6/1
  Gain5/1 -> Add3/1
  Gain6/1 -> Add3/2
  Product2/1 -> Gain3/1
  Product3/1 -> Gain4/1
  Gain3/1 -> Add2/1
  Gain4/1 -> Add2/2
  Gain2/1 -> Add1/2
  Gain1/1 -> Add1/1
  Product1/1 -> Gain2/1
  Product/1 -> Gain1/1
  Math Function3/1 -> Add/4
  Math Function2/1 -> Add/3
  Math Function1/1 -> Add/2
  Math Function/1 -> Add/1
  Add7/1 -> Vector Concatenate2/3  "dcm33"
  Add8/1 -> Vector Concatenate2/2  "dcm23"
  Add3/1 -> Vector Concatenate2/1  "dcm13"
  Add2/1 -> Vector Concatenate1/3  "dcm32"
  Add6/1 -> Vector Concatenate1/2  "dcm22"
  Add4/1 -> Vector Concatenate1/1  "dcm12"
  Add5/1 -> Vector Concatenate/3  "dcm31"
  Add1/1 -> Vector Concatenate/2  "dcm21"
  Add/1 -> Vector Concatenate/1  "dcm11"
  Vector Concatenate1/1 -> Vector Concatenate3/2
  Vector Concatenate2/1 -> Vector Concatenate3/3
  Vector Concatenate/1 -> Vector Concatenate3/1
  Vector Concatenate3/1 -> T12/1
  Demux/4 -> Product3/2, Product11/2, Math Function11/1, Product5/2, Math Function3/1, Product1/2, Product9/2, Product7/2, Math Function7/1  "q4 / q0"
  Demux/3 -> Math Function2/1, Product1/1, Product8/2, Product7/1, Math Function6/1, Product10/2, Math Function10/1, Product4/2, Product2/2  "q3"
  Demux/2 -> Math Function1/1, Product/2, Product9/1, Product6/2, Math Function5/1, Math Function9/1, Product10/1, Product5/1, Product2/1  "q2"
  Demux/1 -> Product6/1, Math Function4/1, Math Function8/1, Product11/1, Product4/1, Product3/1, Math Function/1, Product/1, Product8/1  "q1"
  q12/1 -> Demux/1

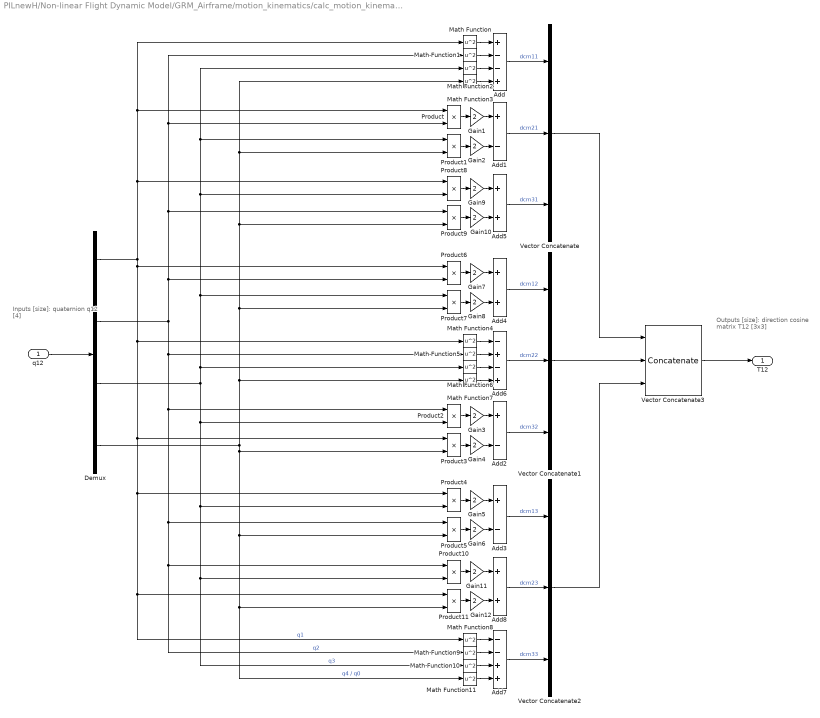
== system PILnewH/Non-linear Flight Dynamic Model/GRM_Airframe/motion_kinematics/calc_motion_kinematics/calc_transformation_matrix/T12_from_q2 ==
  note: Inputs [size]:
      |
      | quaternion q12 [4]
  note: Outputs [size]:
      |
      | direction cosine matrix T12 [3x3]
  q12 : Inport  PortDimensions=4
  Add : Sum  Inputs=+--+
  Add1 : Sum  Inputs=+-
  Add2 : Sum  Inputs=+-
  Add3 : Sum  Inputs=+-
  Add4 : Sum
  Add5 : Sum
  Add6 : Sum  Inputs=-+-+
  Add7 : Sum  Inputs=--++
  Add8 : Sum
  Demux : Demux
  Gain{1..12} (12 alike) : Gain  Gain=2
  Math Function{,1..11} (12 alike) : Math  Operator=square  SignedPower=on  SaturateOnIntegerOverflow=on
  Product{,1..11} (12 alike) : Product
  Vector Concatenate : Concatenate  NumInputs=3
  Vector Concatenate1 : Concatenate  NumInputs=3
  Vector Concatenate2 : Concatenate  NumInputs=3
  Vector Concatenate3 : Concatenate  NumInputs=3  Mode=Multidimensional array  ConcatenateDimension=2
  T12 : Outport  PortDimensions=[3 3]  VectorParamsAs1DForOutWhenUnconnected=off
  wires:
  Product10/1 -> Gain11/1
  Product11/1 -> Gain12/1
  Gain11/1 -> Add8/1
  Gain12/1 -> Add8/2
  Math Function8/1 -> Add7/1
  Math Function9/1 -> Add7/2
  Math Function11/1 -> Add7/4
  Math Function10/1 -> Add7/3
  Math Function4/1 -> Add6/1
  Math Function5/1 -> Add6/2
  Math Function7/1 -> Add6/4
  Math Function6/1 -> Add6/3
  Product8/1 -> Gain9/1
  Product9/1 -> Gain10/1
  Gain9/1 -> Add5/1
  Gain10/1 -> Add5/2
  Product6/1 -> Gain7/1
  Product7/1 -> Gain8/1
  Gain7/1 -> Add4/1
  Gain8/1 -> Add4/2
  Product4/1 -> Gain5/1
  Product5/1 -> Gain6/1
  Gain5/1 -> Add3/1
  Gain6/1 -> Add3/2
  Product2/1 -> Gain3/1
  Product3/1 -> Gain4/1
  Gain3/1 -> Add2/1
  Gain4/1 -> Add2/2
  Gain2/1 -> Add1/2
  Gain1/1 -> Add1/1
  Product1/1 -> Gain2/1
  Product/1 -> Gain1/1
  Math Function3/1 -> Add/4
  Math Function2/1 -> Add/3
  Math Function1/1 -> Add/2
  Math Function/1 -> Add/1
  Add7/1 -> Vector Concatenate2/3  "dcm33"
  Add8/1 -> Vector Concatenate2/2  "dcm23"
  Add3/1 -> Vector Concatenate2/1  "dcm13"
  Add2/1 -> Vector Concatenate1/3  "dcm32"
  Add6/1 -> Vector Concatenate1/2  "dcm22"
  Add4/1 -> Vector Concatenate1/1  "dcm12"
  Add5/1 -> Vector Concatenate/3  "dcm31"
  Add1/1 -> Vector Concatenate/2  "dcm21"
  Add/1 -> Vector Concatenate/1  "dcm11"
  Vector Concatenate1/1 -> Vector Concatenate3/2
  Vector Concatenate2/1 -> Vector Concatenate3/3
  Vector Concatenate/1 -> Vector Concatenate3/1
  Vector Concatenate3/1 -> T12/1
  Demux/4 -> Product3/2, Product11/2, Math Function11/1, Product5/2, Math Function3/1, Product1/2, Product9/2, Product7/2, Math Function7/1  "q4 / q0"
  Demux/3 -> Math Function2/1, Product1/1, Product8/2, Product7/1, Math Function6/1, Product10/2, Math Function10/1, Product4/2, Product2/2  "q3"
  Demux/2 -> Math Function1/1, Product/2, Product9/1, Product6/2, Math Function5/1, Math Function9/1, Product10/1, Product5/1, Product2/1  "q2"
  Demux/1 -> Product6/1, Math Function4/1, Math Function8/1, Product11/1, Product4/1, Product3/1, Math Function/1, Product/1, Product8/1  "q1"
  q12/1 -> Demux/1

== system PILnewH/Non-linear Flight Dynamic Model/GRM_Airframe/motion_kinematics/calc_motion_kinematics/calc_transformation_matrix/conjugate_quaternion ==
  note: Outputs [size]:
      |
      | q_conj [4]
  note: Inputs [size]:
      |
      | q [4]
  q : Inport
  Demux : Demux  Outputs=[3;1]
  Gain1 : Gain  Gain=-1
  Vector Concatenate : Concatenate
  q_conj : Outport  VectorParamsAs1DForOutWhenUnconnected=off
  wires:
  Demux/2 -> Vector Concatenate/2
  Gain1/1 -> Vector Concatenate/1
  Demux/1 -> Gain1/1
  Vector Concatenate/1 -> q_conj/1
  q/1 -> Demux/1

== system PILnewH/Non-linear Flight Dynamic Model/GRM_Airframe/motion_kinematics/calc_motion_kinematics/calc_transformation_matrix/q31_from_q32_mul_q1 ==
  note: Outputs [size]:
      |
      | quaternion q31 [4]
  note: Inputs [size]:
      |
      | quaternion q32 [4]
      | quaternion q21 [4]
  q32 : Inport
  q21 : Inport  Port=2
  Add : Sum  Inputs=++++
  Constant : Constant
  Constant1 : Constant  Value=-1
  Demux1 : Demux
  Product{,1..4} (5 alike) : Product
  Product8 : Product  Multiplication=Matrix(*)
  Q_1 : Constant  Value=[0 0 0 1; 0 0 1 0; 0 -1 0 0; -1 0 0 0]
  Q_2 : Constant  Value=[0 0 -1 0; 0 0 0 1; 1 0 0 0; 0 -1 0 0]
  Q_3 : Constant  Value=[0 1 0 0; -1 0 0 0; 0 0 0 1; 0 0 -1 0]
  Q_4 : Constant  Value=[1 0 0 0; 0 1 0 0; 0 0 1 0; 0 0 0 1]
  Selector : Selector  IndexMode=Zero-based  InputPortWidth=4  IndexOptions=Index vector (dialog)  Indices=3  OutputSizes=1
  Switch : Switch
  normalize_quaternion : Subsystem
      mask help: normalize a quaternion
      mask Help:
      | Name:
      | 
      |     normalize_quaternion
      | 
      | Description:
      | 
      |     This block normalizes the quaternion q21. It should be used as a
      |     safety measure when computing quaternions.
      | 
      | Inputs  [size] [data type] [unit]:
      | 
      |     attitude quaternion q21  [4] [double] [-]
      | 
      | Outputs  [size] [data type] [unit]:
      | 
      |     normalized attitude quaternion q21  [4] [double] [-]
      mask Display: disp (' norm(q)')
  q31 : Outport  VectorParamsAs1DForOutWhenUnconnected=off
  wires:
  Switch/1 -> Product4/2
  Constant/1 -> Switch/1
  Constant1/1 -> Switch/3
  Product4/1 -> q31/1
  Selector/1 -> Switch/2
  normalize_quaternion/1(q_normalized) -> Selector/1, Product4/1
  Product8/1 -> normalize_quaternion/1(q)
  q32/1 -> Demux1/1
  Add/1 -> Product8/1  "Q(q32)"
  Product3/1 -> Add/4
  Product2/1 -> Add/3
  Product1/1 -> Add/2
  Product/1 -> Add/1
  Q_4/1 -> Product3/1
  Q_3/1 -> Product2/1
  Q_2/1 -> Product1/1
  Q_1/1 -> Product/1
  Demux1/4 -> Product3/2  "q4"
  Demux1/3 -> Product2/2  "q3"
  Demux1/2 -> Product1/2  "q2"
  Demux1/1 -> Product/2  "q1"
  q21/1 -> Product8/2

== system PILnewH/Non-linear Flight Dynamic Model/GRM_Airframe/motion_kinematics/calc_motion_kinematics/calc_transformation_matrix/q31_from_q32_mul_q2 ==
  note: Outputs [size]:
      |
      | quaternion q31 [4]
  note: Inputs [size]:
      |
      | quaternion q32 [4]
      | quaternion q21 [4]
  q32 : Inport
  q21 : Inport  Port=2
  Add : Sum  Inputs=++++
  Constant : Constant
  Constant1 : Constant  Value=-1
  Demux1 : Demux
  Product{,1..4} (5 alike) : Product
  Product8 : Product  Multiplication=Matrix(*)
  Q_1 : Constant  Value=[0 0 0 1; 0 0 1 0; 0 -1 0 0; -1 0 0 0]
  Q_2 : Constant  Value=[0 0 -1 0; 0 0 0 1; 1 0 0 0; 0 -1 0 0]
  Q_3 : Constant  Value=[0 1 0 0; -1 0 0 0; 0 0 0 1; 0 0 -1 0]
  Q_4 : Constant  Value=[1 0 0 0; 0 1 0 0; 0 0 1 0; 0 0 0 1]
  Selector : Selector  IndexMode=Zero-based  InputPortWidth=4  IndexOptions=Index vector (dialog)  Indices=3  OutputSizes=1
  Switch : Switch
  normalize_quaternion : Subsystem
      mask help: normalize a quaternion
      mask Help:
      | Name:
      | 
      |     normalize_quaternion
      | 
      | Description:
      | 
      |     This block normalizes the quaternion q21. It should be used as a
      |     safety measure when computing quaternions.
      | 
      | Inputs  [size] [data type] [unit]:
      | 
      |     attitude quaternion q21  [4] [double] [-]
      | 
      | Outputs  [size] [data type] [unit]:
      | 
      |     normalized attitude quaternion q21  [4] [double] [-]
      mask Display: disp (' norm(q)')
  q31 : Outport  VectorParamsAs1DForOutWhenUnconnected=off
  wires:
  Switch/1 -> Product4/2
  Constant/1 -> Switch/1
  Constant1/1 -> Switch/3
  Product4/1 -> q31/1
  Selector/1 -> Switch/2
  normalize_quaternion/1(q_normalized) -> Selector/1, Product4/1
  Product8/1 -> normalize_quaternion/1(q)
  q32/1 -> Demux1/1
  Add/1 -> Product8/1  "Q(q32)"
  Product3/1 -> Add/4
  Product2/1 -> Add/3
  Product1/1 -> Add/2
  Product/1 -> Add/1
  Q_4/1 -> Product3/1
  Q_3/1 -> Product2/1
  Q_2/1 -> Product1/1
  Q_1/1 -> Product/1
  Demux1/4 -> Product3/2  "q4"
  Demux1/3 -> Product2/2  "q3"
  Demux1/2 -> Product1/2  "q2"
  Demux1/1 -> Product/2  "q1"
  q21/1 -> Product8/2

== system PILnewH/Non-linear Flight Dynamic Model/GRM_Airframe/motion_kinematics/calc_motion_kinematics/calc_transformation_matrix/q31_from_q32_mul_q21 ==
  note: Outputs [size]:
      |
      | quaternion q31 [4]
  note: Inputs [size]:
      |
      | quaternion q32 [4]
      | quaternion q21 [4]
  q32 : Inport
  q21 : Inport  Port=2
  Add : Sum  Inputs=++++
  Constant : Constant
  Constant1 : Constant  Value=-1
  Demux1 : Demux
  Product{,1..4} (5 alike) : Product
  Product8 : Product  Multiplication=Matrix(*)
  Q_1 : Constant  Value=[0 0 0 1; 0 0 1 0; 0 -1 0 0; -1 0 0 0]
  Q_2 : Constant  Value=[0 0 -1 0; 0 0 0 1; 1 0 0 0; 0 -1 0 0]
  Q_3 : Constant  Value=[0 1 0 0; -1 0 0 0; 0 0 0 1; 0 0 -1 0]
  Q_4 : Constant  Value=[1 0 0 0; 0 1 0 0; 0 0 1 0; 0 0 0 1]
  Selector : Selector  IndexMode=Zero-based  InputPortWidth=4  IndexOptions=Index vector (dialog)  Indices=3  OutputSizes=1
  Switch : Switch
  normalize_quaternion : Subsystem
      mask help: normalize a quaternion
      mask Help:
      | Name:
      | 
      |     normalize_quaternion
      | 
      | Description:
      | 
      |     This block normalizes the quaternion q21. It should be used as a
      |     safety measure when computing quaternions.
      | 
      | Inputs  [size] [data type] [unit]:
      | 
      |     attitude quaternion q21  [4] [double] [-]
      | 
      | Outputs  [size] [data type] [unit]:
      | 
      |     normalized attitude quaternion q21  [4] [double] [-]
      mask Display: disp (' norm(q)')
  q31 : Outport  VectorParamsAs1DForOutWhenUnconnected=off
  wires:
  Switch/1 -> Product4/2
  Constant/1 -> Switch/1
  Constant1/1 -> Switch/3
  Product4/1 -> q31/1
  Selector/1 -> Switch/2
  normalize_quaternion/1(q_normalized) -> Selector/1, Product4/1
  Product8/1 -> normalize_quaternion/1(q)
  q32/1 -> Demux1/1
  Add/1 -> Product8/1  "Q(q32)"
  Product3/1 -> Add/4
  Product2/1 -> Add/3
  Product1/1 -> Add/2
  Product/1 -> Add/1
  Q_4/1 -> Product3/1
  Q_3/1 -> Product2/1
  Q_2/1 -> Product1/1
  Q_1/1 -> Product/1
  Demux1/4 -> Product3/2  "q4"
  Demux1/3 -> Product2/2  "q3"
  Demux1/2 -> Product1/2  "q2"
  Demux1/1 -> Product/2  "q1"
  q21/1 -> Product8/2

== system PILnewH/Non-linear Flight Dynamic Model/GRM_Airframe/motion_kinematics/calc_motion_kinematics/earth_rotation/earth_rotation_rate ==
  Constant6 : Constant  Value=0
  Constant7 : Constant  Value=c_rot
  Constant8 : Constant  Value=0
  Constant9 : Constant  Value=flag_I_rot
  Switch : Switch  Criteria=u2 > Threshold
  Vector Concatenate : Concatenate  NumInputs=3
  Vector Concatenate1 : Concatenate  NumInputs=3
  wIEE : Outport  VectorParamsAs1DForOutWhenUnconnected=off
  wires:
  Switch/1 -> wIEE/1  "wIEE"
  Constant6/1 -> Vector Concatenate/2, Vector Concatenate/1
  Constant9/1 -> Switch/2
  Vector Concatenate/1 -> Switch/1  "wIEE"
  Constant7/1 -> Vector Concatenate/3
  Vector Concatenate1/1 -> Switch/3  "wIEE"
  Constant8/1 -> Vector Concatenate1/1, Vector Concatenate1/3, Vector Concatenate1/2
